simulink model "lab2_part2"  (R2022a)
settings: Solver=VariableStepAuto  StartTime=0.0  StopTime=30  RelTol=10e-10  AbsTol=10e-10
settings Model: Creator=yuans  LastModifiedBy=yuans

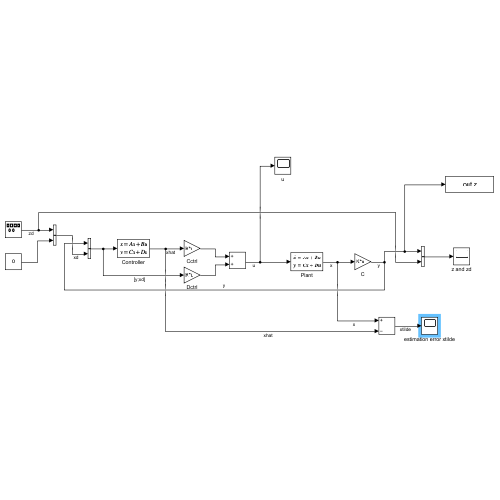
[thumbnail: Simulink's stored preview of the top-level diagram]
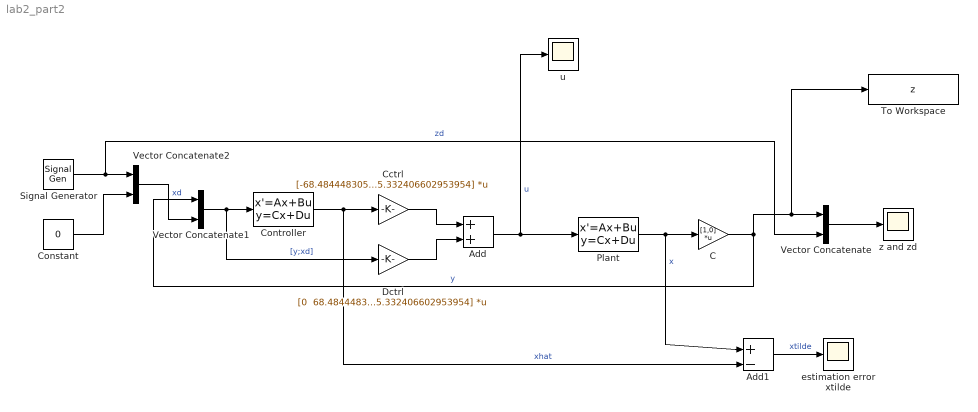
== system lab2_part2 ==
  Add : Sum
  Add1 : Sum  Inputs=+|-
  C : Gain  Gain=[1,0]  Multiplication=Matrix(K*u)
  Cctrl : Gain  Gain="[-68.484448305821033  -5.332406602953954]"  Multiplication=Matrix(K*u)
  Constant : Constant  Value=0
  Controller : StateSpace  A=|  B=|  C=[1 0;0 1]  D=[0 0 0; 0 0 0]  InitialCondition=0  ParameterTunability=Unconstrained
      A=|
      | [  -27.2122762148338   1.0000000000000;
      |   -196.0169281990568  -24.0000000000000]
      B=|
      | [27.2122762148338                   0                   0;
      |    52.0169281990568   144.0000000000000   11.2122762148338]
  Dctrl : Gain  Gain="[0  68.484448305821033   5.332406602953954]"  Multiplication=Matrix(K*u)
  Plant : StateSpace  A=[0 1;0 -12.787723785166239]  B=[0;2.102667153818049]  C=[1 0;0 1]  D=[0;0]  InitialCondition=0  ParameterTunability=Unconstrained
  Signal Generator : SignalGenerator  WaveForm=square  Amplitude=0.03  Frequency=0.1
  To Workspace : ToWorkspace  VariableName=z  SaveFormat=Timeseries  SampleTime=-1
  Vector Concatenate : Concatenate
  Vector Concatenate1 : Concatenate
  Vector Concatenate2 : Concatenate
  estimation error xtilde : Scope
  u : Scope
  z and zd : Scope
  wires:
  Plant/1 -> Add1/1, C/1  "x"
  Add/1 -> Plant/1, u/1  "u"
  Cctrl/1 -> Add/1
  Dctrl/1 -> Add/2
  Controller/1 -> Add1/2, Cctrl/1  "xhat"
  Add1/1 -> estimation error xtilde/1  "xtilde"
  Vector Concatenate1/1 -> Dctrl/1, Controller/1  "[y;xd]"
  Vector Concatenate2/1 -> Vector Concatenate1/2  "xd"
  C/1 -> To Workspace/1, Vector Concatenate/1, Vector Concatenate1/1  "y"
  Signal Generator/1 -> Vector Concatenate/2, Vector Concatenate2/1  "zd"
  Constant/1 -> Vector Concatenate2/2
  Vector Concatenate/1 -> z and zd/1
